simulink model "testEncoderRead"  (R2018b)
settings: Solver=FixedStepDiscrete  StartTime=0.0  StopTime=10.0  FixedStep=.1  RelTol=1e-3  EnableMultiTasking=on
libraries: arduinolib x3
settings Model: ExtModeTrigDuration=2  Creator=KSURCT General  LastModifiedBy=KSURCT General
settings OptimizationCC: EnhancedBackFolding=on  PassReuseOutputArgsAs=Individual arguments  MaxStackSize=64  OptimizeBlockOrder=speed  DifferentSizesBufferReuse=on  OptimizationCustomize=off
settings DebuggingCC: ParameterTunabilityLossMsg=error
settings HardwareCC: ProdBitPerPointer=32  ProdBitPerSizeT=32  ProdBitPerPtrDiffT=32  ProdLargestAtomicInteger=Long  ProdLargestAtomicFloat=Double  ProdWordSize=32  ProdHWDeviceType=ARM Compatible->ARM Cortex
settings SFSimCC: MATLABDynamicMemAlloc=off
settings RTWCC: SystemTargetFile=ert.tlc  HardwareBoard=Arduino Due  TemplateMakefile=ert_default_tmf  GenerateReport=on  Toolchain=Arduino ARM  BuildConfiguration=Faster Runs  IncludeHyperlinkInReport=on  LaunchReport=on  GenerateTraceInfo=on  GenerateTraceReport=on  GenerateTraceReportSl=on  GenerateTraceReportSf=on  GenerateTraceReportEml=on
settings CodeAppCC: ForceParamTrailComments=on  IgnoreCustomStorageClasses=off  OperatorAnnotations=on  SimulinkDataObjDesc=on  SFDataObjDesc=on  InsertBlockDesc=on
settings ERTTargetCC: SupportContinuousTime=on  SupportVariableSizeSignals=on

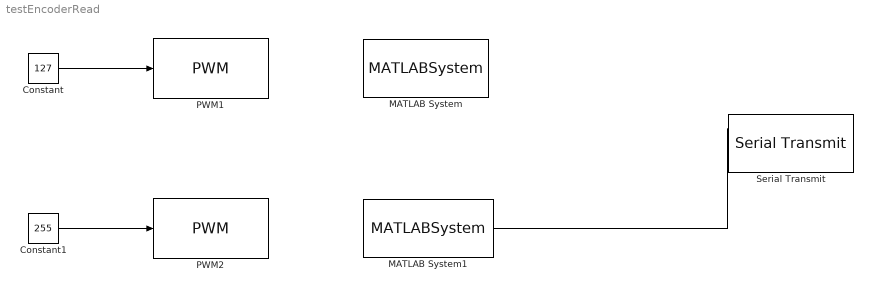
== system testEncoderRead ==
  Constant : Constant  Value=127
  Constant1 : Constant  Value=255
  MATLAB System : MATLABSystem  System=EncoderRead  pinA=int8(12)  pinB=int8(11)  id=int8(1)  SampleTime=-1
      mask Type: EncoderRead
      mask Display:
      | disp('Source');
      | port_label('output',1,'ticks');
  MATLAB System1 : MATLABSystem  System=EncoderRead  pinA=int8(11)  pinB=int8(10)  id=int8(0)  SampleTime=-1
      mask Type: EncoderRead
      mask Display:
      | disp('Source');
      | port_label('output',1,'ticks');
  PWM1 : arduinolib/PWM  pinNumber=4  EnableInputFrequency=off  InitialFrequency=2000  InitialDutyCycle=0  NotificationType=None  blockPlatform=arduino
  PWM2 : arduinolib/PWM  pinNumber=2  EnableInputFrequency=off  InitialFrequency=2000  InitialDutyCycle=0  NotificationType=None  blockPlatform=arduino
  Serial Transmit : arduinolib/Serial Transmit  portNumber=0  sendmode=println  label=right >>  sendformat=Decimal  floatprecision=2  blockPlatform=arduino
      settings: SourceProductName=Simulink Support Package for Arduino Hardware
  wires:
  Constant/1 -> PWM1/1
  Constant1/1 -> PWM2/1
  MATLAB System1/1 -> ?
